simulink model "Multilevel_inverter_topology_based_on_series"  (Simulink 8.4)
settings: Solver=ode45  StartTime=0.0  StopTime=0.5  MaxStep=.00001  RelTol=1e-3
libraries: powerlib x11, simulink x4, powerlib_meascontrol x1
settings Model: Creator=Muruganandham  LastModifiedBy=SELVA
settings ConfigurationSet: Description=SimMechanics 2G

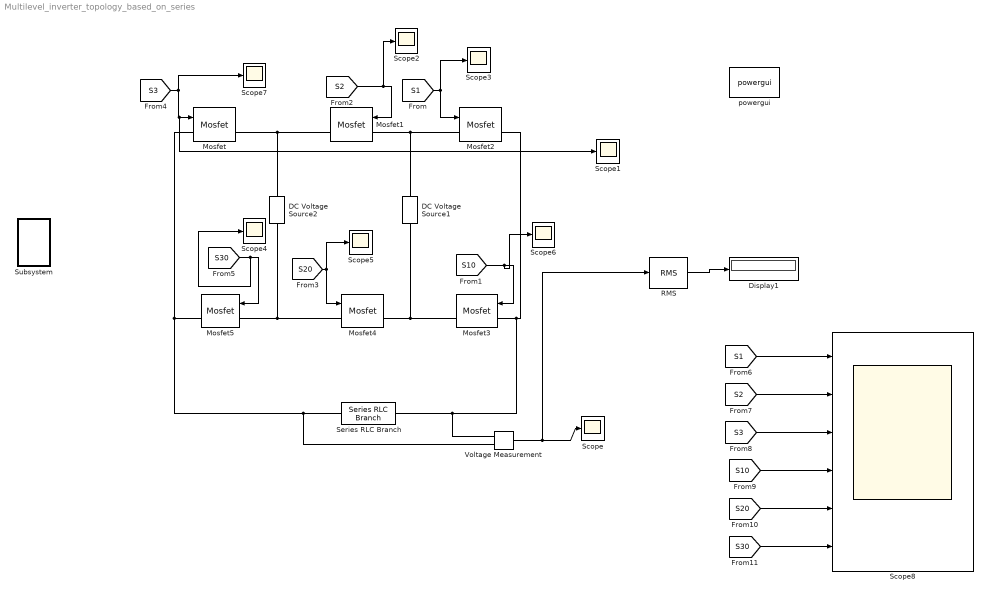
== system Multilevel_inverter_topology_based_on_series ==
  DC Voltage Source1 : powerlib/Electrical Sources/DC Voltage Source  Amplitude=100  Measurements=None
  DC Voltage Source2 : powerlib/Electrical Sources/DC Voltage Source  Amplitude=100  Measurements=None
  Display1 : Display
  Mosfet{,1..5} (6 alike) : powerlib/Power Electronics/Mosfet  Ron=0.1  Lon=0  Rd=0.01  Vfd=0  IC=0  Rs=1e5  Cs=inf  Measurements=on
  RMS : powerlib_meascontrol/Measurements/RMS  TrueRMS=on  Freq=50  RMSInit=120  Ts=0
  Scope{,1..7} (8 alike) : Scope
      Scope settings: YMin=-200  YMax=200  SaveName=bh
      Scope1 settings: YMin=-200  YMax=200  SaveName=bh1
      Scope2 settings: YMin=-200  YMax=200  SaveName=bh2
      Scope3 settings: YMin=-1  YMax=1.5  SaveName=bh3
      Scope4 settings: YMin=-200  YMax=200  SaveName=bh4
      Scope5 settings: YMin=-200  YMax=200  SaveName=bh5
      Scope6 settings: YMin=-1  YMax=1.5  SaveName=bh6
      Scope7 settings: YMin=-1  YMax=1.5  SaveName=bh7
  Scope8 : Scope  NumInputPorts=6
      settings: YMin=-0.5~-0.5~-0.5~-0.5~-0.5~-0.5  YMax=1.5~1.5~1.5~1.5~1.5~1.5  SaveName=bh8
  Series RLC Branch : powerlib/Elements/Series RLC Branch  LConnTagsString=__new0  RConnTagsString=__new0  BranchType=R  Resistance=100  Inductance=1e-3  SetiL0=off  InitialCurrent=0  Capacitance=1e-6  Setx0=off  InitialVoltage=0  Measurements=None
  Subsystem : Subsystem  mask{fc=1000, m=1}
      mask prompts: fc "Switching frequency"; m "modulation index"
  Voltage Measurement : powerlib/Measurements/Voltage Measurement  PhasorSimulation=off  OutputType=Complex  PSBequivalent=0
  powergui : powerlib/powergui  Priority=1  SimulationMode=Continuous  SolverType=Tustin  SampleTime=50e-6  frequency=60  SPID=off  DisableSnubberDevices=off  DisableRonSwitches=off  DisableVfSwitches=off  SwTol=0  DisplayEquations=off  Interpol=off  methode=off  Ts=0  frequencyindice=0  Pbase=100e6  ErrMax=1e-4  Iterations=50  UnitsV=kV  UnitsW=MW  FunctionMessages=off  echomessages=off  HookPort=off  EnableUseOfTLC=off  x0status=blocks  RestoreLinks=warning  ResistiveCurrentMeasurement=off  Frange=[0:2:500]  Ylog=off  Xlog=on  ShowGrid=off  save=off  variable=ZData  structure=bh  ZoomFFT=off  StartTime=0.0  cycles=1  DisplayStyle=1  fundamental=50  FreqAxis=off  MaxFrequency=1000  frequencyindicesteady=1  RmsSteady=1  display=off
  wires:
  [S2] -> Mosfet1/1, Scope2/1
  [S20] -> Mosfet4/1, Scope5/1
  [S3] -> Mosfet/1, Scope1/1, Scope7/1
  [S30] -> Mosfet5/1, Scope4/1
  Voltage Measurement/1 -> RMS/1, Scope/1
  RMS/1 -> Display1/1
  [S10] -> Mosfet3/1, Scope6/1
  [S1] -> Mosfet2/1, Scope3/1
  [S30] -> Scope8/6
  [S10] -> Scope8/4
  [S3] -> Scope8/3
  [S20] -> Scope8/5
  [S2] -> Scope8/2
  [S1] -> Scope8/1
  connections:
  DC Voltage Source2/LConn1 -- Mosfet1/RConn1 -- Mosfet/RConn1
  DC Voltage Source1/RConn1 -- Mosfet2/LConn1 -- Mosfet1/LConn1
  DC Voltage Source2/RConn1 -- Mosfet4/LConn1 -- Mosfet5/LConn1
  DC Voltage Source1/LConn1 -- Mosfet4/RConn1 -- Mosfet3/RConn1
  Series RLC Branch/LConn1 -- Mosfet5/RConn1 -- Mosfet/LConn1 -- Voltage Measurement/LConn2
  Series RLC Branch/RConn1 -- Mosfet3/LConn1 -- Mosfet2/RConn1 -- Voltage Measurement/LConn1

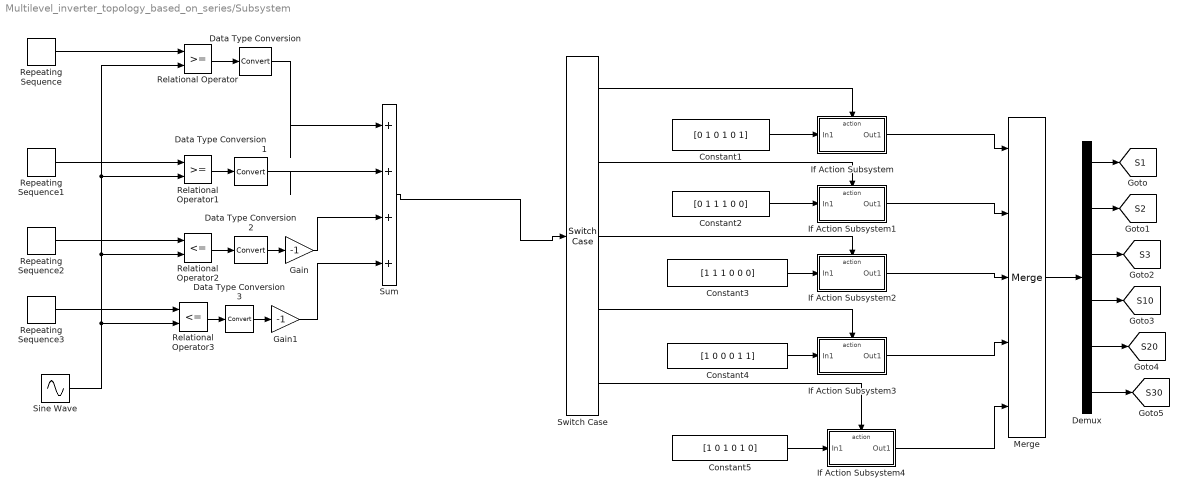
== system Multilevel_inverter_topology_based_on_series/Subsystem ==
  Constant1 : Constant  Value=[0 1 0 1 0 1]
  Constant2 : Constant  Value=[0 1 1 1 0 0]
  Constant3 : Constant  Value=[1 1 1 0 0 0]
  Constant4 : Constant  Value=[1 0 0 0 1 1]
  Constant5 : Constant  Value=[1 0 1 0 1 0]
  Data Type Conversion{,1..3} (4 alike) : DataTypeConversion
  Demux : Demux  Outputs=6
  Gain : Gain  Gain=-1
  Gain1 : Gain  Gain=-1
  If Action Subsystem : Subsystem  TreatAsAtomicUnit=on
  If Action Subsystem1 : Subsystem  TreatAsAtomicUnit=on
  If Action Subsystem2 : Subsystem  TreatAsAtomicUnit=on
  If Action Subsystem3 : Subsystem  TreatAsAtomicUnit=on
  If Action Subsystem4 : Subsystem  TreatAsAtomicUnit=on
  Merge : Merge  Inputs=5
  Relational Operator : RelationalOperator  OutDataTypeStr=boolean
  Relational Operator1 : RelationalOperator  OutDataTypeStr=boolean
  Relational Operator2 : RelationalOperator  Operator=<=  OutDataTypeStr=boolean
  Relational Operator3 : RelationalOperator  Operator=<=  OutDataTypeStr=boolean
  Repeating Sequence : simulink/Sources/Repeating Sequence  rep_seq_t="[0 (1/fc)/2  (1/fc)]"  rep_seq_y=[1 2 1]
  Repeating Sequence1 : simulink/Sources/Repeating Sequence  rep_seq_t="[0 (1/fc)/2  (1/fc)]"  rep_seq_y=[1 0 1]
  Repeating Sequence2 : simulink/Sources/Repeating Sequence  rep_seq_t="[0 (1/fc)/2  (1/fc)]"  rep_seq_y=[-1 0 -1]
  Repeating Sequence3 : simulink/Sources/Repeating Sequence  rep_seq_t="[0 (1/fc)/2  (1/fc)]"  rep_seq_y=[-1 -2 -1]
  Sine Wave : Sin  Amplitude=2*m  Frequency=2*pi*50  SampleTime=0
  Sum : Sum  Inputs=|++++
  Switch Case : SwitchCase  CaseConditions={-2 -1 0 1 2}  ShowDefaultCase=off
  tag scope: S10=global, S1=global, S20=global, S2=global, S30=global, S3=global
  wires:
  Switch Case/5 -> If Action Subsystem4/Action
  Switch Case/4 -> If Action Subsystem3/Action
  Switch Case/3 -> If Action Subsystem2/Action
  Switch Case/2 -> If Action Subsystem1/Action
  Switch Case/1 -> If Action Subsystem/Action
  Constant1/1 -> If Action Subsystem/1(In1)
  Constant2/1 -> If Action Subsystem1/1(In1)
  Constant3/1 -> If Action Subsystem2/1(In1)
  Constant4/1 -> If Action Subsystem3/1(In1)
  Constant5/1 -> If Action Subsystem4/1(In1)
  If Action Subsystem/1(Out1) -> Merge/1
  If Action Subsystem1/1(Out1) -> Merge/2
  If Action Subsystem2/1(Out1) -> Merge/3
  If Action Subsystem3/1(Out1) -> Merge/4
  If Action Subsystem4/1(Out1) -> Merge/5
  Merge/1 -> Demux/1
  Demux/2 -> [S2]
  Demux/3 -> [S3]
  Demux/4 -> [S10]
  Demux/5 -> [S20]
  Demux/6 -> [S30]
  Relational Operator/1 -> Data Type Conversion/1
  Relational Operator1/1 -> Data Type Conversion1/1
  Gain/1 -> Sum/3
  Gain1/1 -> Sum/4
  Sum/1 -> Switch Case/1
  Repeating Sequence/1 -> Relational Operator/1
  Repeating Sequence1/1 -> Relational Operator1/1
  Repeating Sequence2/1 -> Relational Operator2/1
  Repeating Sequence3/1 -> Relational Operator3/1
  Sine Wave/1 -> Relational Operator1/2, Relational Operator/2, Relational Operator2/2, Relational Operator3/2
  Relational Operator2/1 -> Data Type Conversion2/1
  Relational Operator3/1 -> Data Type Conversion3/1
  Data Type Conversion/1 -> Sum/1
  Data Type Conversion1/1 -> Sum/2
  Data Type Conversion2/1 -> Gain/1
  Data Type Conversion3/1 -> Gain1/1
  Demux/1 -> [S1]

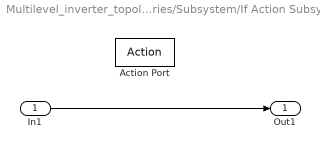
== system Multilevel_inverter_topology_based_on_series/Subsystem/If Action Subsystem ==
  In1 : Inport
  Action Port : ActionPort
  Out1 : Outport
  wires:
  In1/1 -> Out1/1

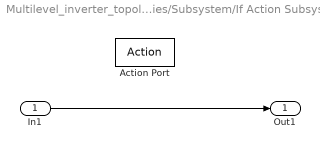
== system Multilevel_inverter_topology_based_on_series/Subsystem/If Action Subsystem1 ==
  In1 : Inport
  Action Port : ActionPort
  Out1 : Outport
  wires:
  In1/1 -> Out1/1

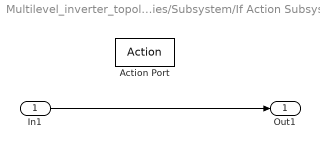
== system Multilevel_inverter_topology_based_on_series/Subsystem/If Action Subsystem2 ==
  In1 : Inport
  Action Port : ActionPort
  Out1 : Outport
  wires:
  In1/1 -> Out1/1

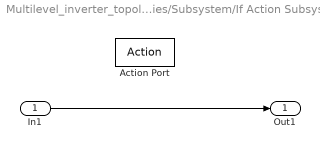
== system Multilevel_inverter_topology_based_on_series/Subsystem/If Action Subsystem3 ==
  In1 : Inport
  Action Port : ActionPort
  Out1 : Outport
  wires:
  In1/1 -> Out1/1

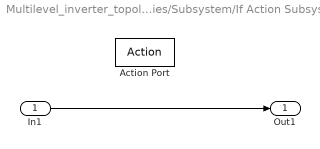
== system Multilevel_inverter_topology_based_on_series/Subsystem/If Action Subsystem4 ==
  In1 : Inport
  Action Port : ActionPort
  Out1 : Outport
  wires:
  In1/1 -> Out1/1
